simulink model "OpenLoop_Test"  (R2023b)
settings: Solver=VariableStepAuto  StartTime=0.0  StopTime=10.0  RelTol=1e-3
libraries: cstblocks x6
settings Model: Creator=PierluigiMeneses  LastModifiedBy=Antonio

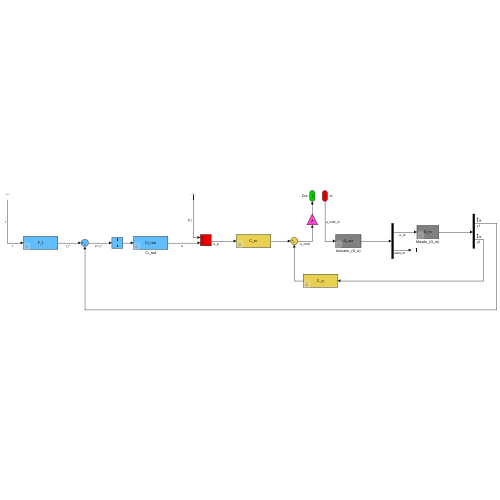
[thumbnail: Simulink's stored preview of the top-level diagram]
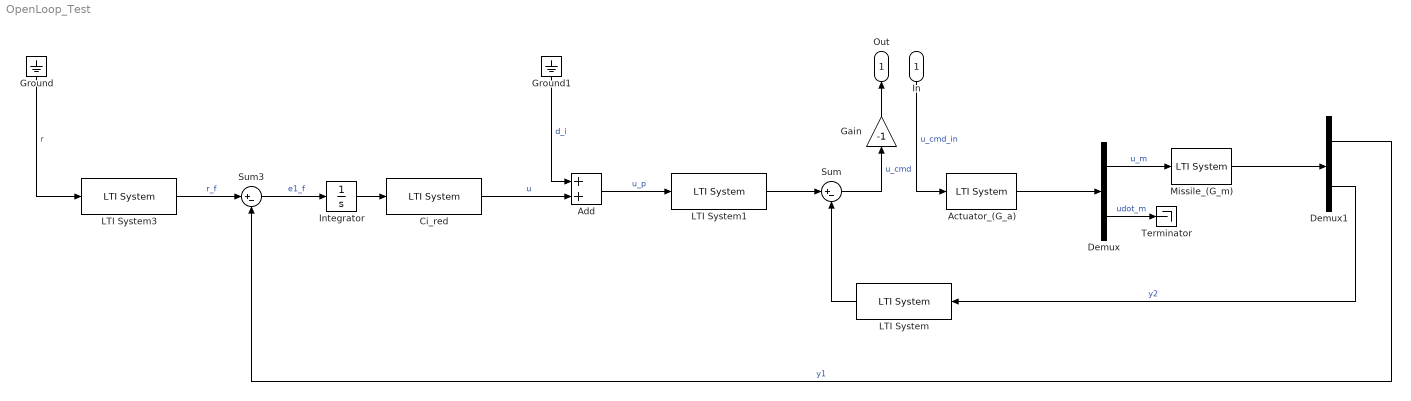
== system OpenLoop_Test ==
  In : Inport
  Actuator_(G_a) : cstblocks/LTI System  sys=G_act  IC=[]  PadeOrder=0
  Add : Sum
  Ci_red : cstblocks/LTI System  sys=Ci_red  IC=[]  PadeOrder=0
  Demux : Demux  Outputs=2
  Demux1 : Demux  Outputs=2
  Gain : Gain  Gain=-1
  Ground : Ground
  Ground1 : Ground
  Integrator : Integrator
  LTI System : cstblocks/LTI System  sys=C_q  IC=[]  PadeOrder=0
  LTI System1 : cstblocks/LTI System  sys=C_sc  IC=[]  PadeOrder=0
  LTI System3 : cstblocks/LTI System  sys=F_f  IC=[]  PadeOrder=0
  Missile_(G_m) : cstblocks/LTI System  sys=G_m  IC=[]  PadeOrder=0
  Sum : Sum  Inputs=|+-
  Sum3 : Sum  Inputs=|+-
  Terminator : Terminator
  Out : Outport
  wires:
  Add/1 -> LTI System1/1  "u_p"
  Demux/1 -> Missile_(G_m)/1  "u_m"
  Demux1/2 -> LTI System/1  "y2"
  LTI System1/1 -> Sum/1
  Actuator_(G_a)/1 -> Demux/1
  Missile_(G_m)/1 -> Demux1/1
  LTI System/1 -> Sum/2
  Demux/2 -> Terminator/1  "udot_m"
  Demux1/1 -> Sum3/2  "y1"
  Ci_red/1 -> Add/2  "u"
  Ground1/1 -> Add/1  "d_i"
  LTI System3/1 -> Sum3/1  "r_f"
  Ground/1 -> LTI System3/1  "r"
  Sum3/1 -> Integrator/1  "e1_f"
  Integrator/1 -> Ci_red/1
  Sum/1 -> Gain/1  "u_cmd"
  In/1 -> Actuator_(G_a)/1  "u_cmd_in"
  Gain/1 -> Out/1
